simulink model "actuators"  (R2026a)
settings: Solver=VariableStepAuto
undefined symbols (not defined in the file): Actuators
libraries: matrix_library x1
settings Model: Creator=arroy  LastModifiedBy=Owner

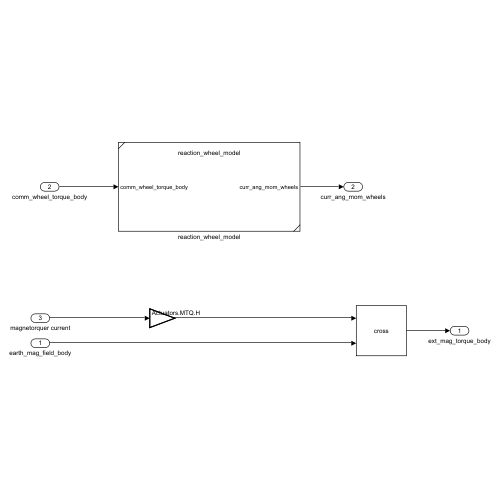
[thumbnail: Simulink's stored preview of the top-level diagram]
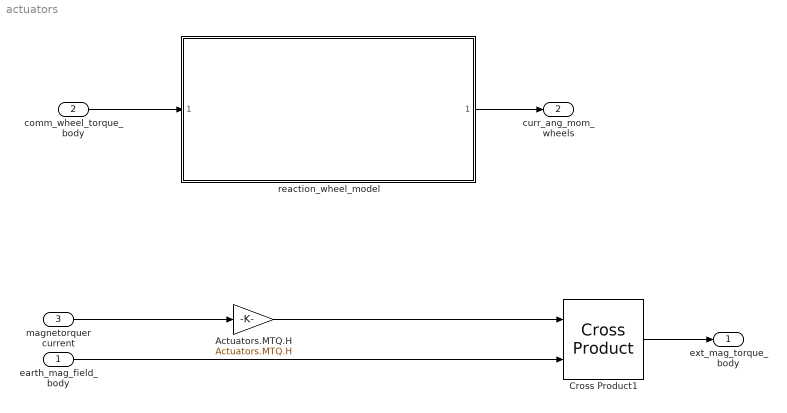
== system actuators ==
  earth_mag_field_body : Inport
  comm_wheel_torque_body : Inport  Port=2
  magnetorquer current : Inport  Port=3
  " Actuators.MTQ.H" : Gain  Gain=Actuators.MTQ.H
  Cross Product1 : matrix_library/Cross Product
  reaction_wheel_model : Subsystem  ReferencedSubsystem=reaction_wheel_model
  ext_mag_torque_body : Outport
  curr_ang_mom_wheels : Outport  Port=2
  wires:
  earth_mag_field_body/1 -> Cross Product1/2
  comm_wheel_torque_body/1 -> reaction_wheel_model/1
  reaction_wheel_model/1 -> curr_ang_mom_wheels/1
  " Actuators.MTQ.H"/1 -> Cross Product1/1
  magnetorquer current/1 -> " Actuators.MTQ.H"/1
  Cross Product1/1 -> ext_mag_torque_body/1
